simulink model "EMB"  (R2019b)
settings: Solver=ode45  StartTime=0.0  StopTime=1  RelTol=1e-3  EnableMultiTasking=on
values from neighbouring files (symbols this model uses):
  a = [1 10501 408092434.54 2.46403599001e+12 1.14030432406e+15 10480.8559648]    [EMB_Variables.mat]
  b = 4e+12    [EMB_Variables.mat]
  c_break = 1000000    [EMB_Variables.mat]
  c_gear = 200000    [EMB_Variables.mat]
  D_Kraft = 0    [EMB_Variables.mat]
  D_Pos = 0    [EMB_Variables.mat]
  d_rot = 0.1    [EMB_Variables.mat]
  d_trans = 0.1    [EMB_Variables.mat]
  i = 113.116658706    [EMB_Variables.mat]
  I_Kraft = 1000    [EMB_Variables.mat]
  I_Pos = 1000    [EMB_Variables.mat]
  J = 1e-05    [EMB_Variables.mat]
  K = 0.02    [EMB_Variables.mat]
  L = 0.001    [EMB_Variables.mat]
  m = 0.1    [EMB_Variables.mat]
  P_Kraft = 10000    [EMB_Variables.mat]
  P_Pos = 10000    [EMB_Variables.mat]
  R = 0.5    [EMB_Variables.mat]
  t0 = 0.1    [EMB_Variables.mat]
  t1 = 0.0025    [EMB_Variables.mat]
  T_abtast = 0.0001    [EMB_Variables.mat]
  x0 = 0.05    [EMB_Variables.mat]
  x_break = 0.0005    [EMB_Variables.mat]
libraries: simulink x3
settings Model: Creator=thomasst  LastModifiedBy=yuxia
settings DataIOCC: SaveFormat=Array  SignalLoggingSaveFormat=ModelDataLogs  ReturnWorkspaceOutputs=off
settings OptimizationCC: LifeSpan=inf
settings DebuggingCC: SolverPrmCheckMsg=warning  MultiTaskDSMMsg=warning  MultiTaskCondExecSysMsg=none  SFUnexpectedBacktrackingDiag=warning  SFNoUnconditionalDefaultTransitionDiag=warning  SFExecutionAtInitializationDiag=none  ArithmeticOperatorsInVariantConditions=warning
settings HardwareCC: ProdBitPerPointer=32  ProdBitPerSizeT=32  ProdBitPerPtrDiffT=32  ProdLargestAtomicFloat=None  ProdIntDivRoundTo=Undefined  ProdEndianess=Unspecified  ProdWordSize=32  ProdHWDeviceType=32-bit Generic
settings ModelReferenceCC: PropagateSignalLabelsOutOfModel=off
settings SFSimCC: SimUseLocalCustomCode=off  CustomCodeUndefinedFunction=UseInterfaceOnly
settings RTWCC: RTWUseLocalCustomCode=off
settings CodeAppCC: StateflowObjectComments=on
settings GRTTargetCC: TargetLangStandard=C89/C90 (ANSI)  GeneratePreprocessorConditionals=Disable all
settings ConfigComp: CovMetricSettings=dw  CovHtmlReporting=on  CovSaveCumulativeToWorkspaceVar=on  CovSaveSingleToWorkspaceVar=on  CovExternalEMLEnable=off

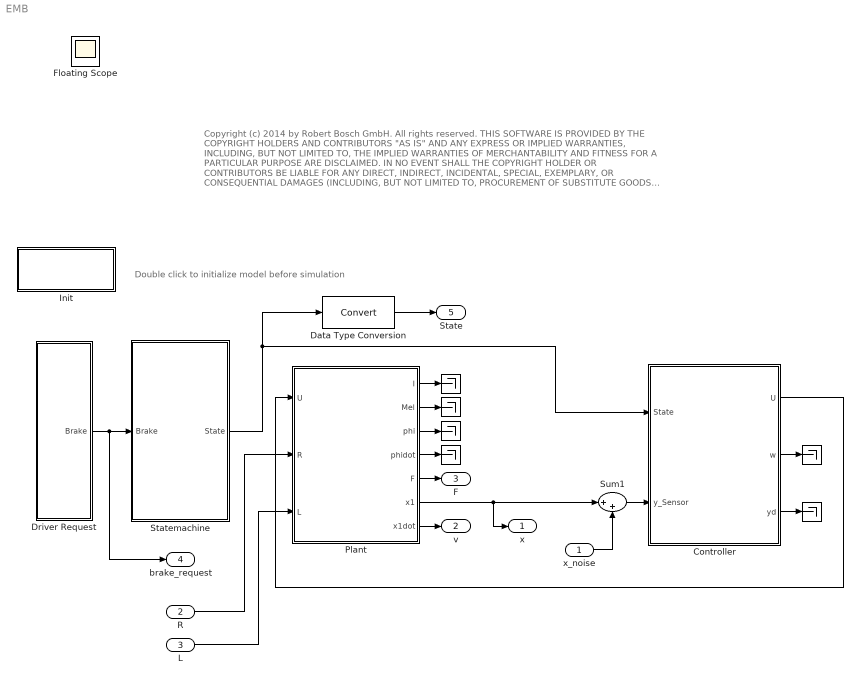
== system EMB ==
  note: Copyright (c) 2014 by Robert Bosch GmbH. All rights reserved.
      |
      | THIS SOFTWARE IS PROVIDED BY THE COPYRIGHT HOLDERS AND CONTRIBUTORS "AS IS"
      | AND ANY EXPRESS OR IMPLIED WARRANTIES, INCLUDING, BUT NOT LIMITED TO, THE IMPLIED
      | WARRANTIES OF MERCHANTABILITY AND FITNESS FOR A PARTICULAR PURPOSE ARE
      | DISCLAIMED. IN NO EVENT SHALL THE COPYRIGHT HOLDER OR CONTRIBUTORS BE LIABLE FOR
      | ANY DIRECT, INDIRECT, INCIDENTAL, SPECIAL, EXEMPLARY, OR CONSEQUENTIAL DAMAGES
      |  (INCLUDING, BUT NOT LIMITED TO, PROCUREMENT OF SUBSTITUTE GOODS OR SERVICES;
      | LOSS OF USE, DATA, OR PROFITS; OR BUSINESS INTERRUPTION) HOWEVER CAUSED AND
      | ON ANY THEORY OF LIABILITY, WHETHER IN CONTRACT, STRICT LIABILITY, OR TORT (INCLUDING
      | NEGLIGENCE OR OTHERWISE) ARISING IN ANY WAY OUT OF THE USE OF THIS SOFTWARE, EVEN
      | IF ADVISED OF THE POSSIBILITY OF SUCH DAMAGE.
      |
      | THE ENTIRE RISK AS TO THE QUALITY AND PERFORMANCE OF THE PROGRAM IS WITH YOU. SHOULD THE PROGRAM PROVE DEFECTIVE,
      | YOU ASSUME THE COST OF ALL NECESSARY SERVICING, REPAIR OR CORRECTION.
      |
      | This is not a model of a Bosch product.
      | This model was originally released in the scope of the ARCH workshop (http://cps-vo.org/group/ARCH).
  note: Double click to initialize model before simulation
  x_noise : Inport
  R : Inport  Port=2
  L : Inport  Port=3
  "  " : Terminator
  "   " : Terminator
  "    " : Terminator
  "      " : Terminator
  "        " : Terminator
  "          " : Terminator
  Controller : Subsystem
  Data Type Conversion : DataTypeConversion
  Driver Request : Subsystem
  Init : Subsystem
      settings: OpenFcn=load('EMB_Variables.mat');
  Plant : Subsystem
  Statemachine : Subsystem
  Sum1 : Sum  Inputs=|++
  x : Outport
  v : Outport  Port=2
  F : Outport  Port=3
  brake_request : Outport  Port=4
  State : Outport  Port=5
  Floating Scope : Scope
  wires:
  Plant/6(x1) -> Sum1/1, x/1
  Plant/3(phi) -> "  "/1
  Plant/4(phidot) -> "   "/1
  Plant/5(F) -> F/1
  Plant/7(x1dot) -> v/1
  x_noise/1 -> Sum1/2
  Plant/2(Mel) -> "    "/1
  Plant/1(I) -> "      "/1
  Sum1/1 -> Controller/2(y_Sensor)
  Controller/1(U) -> Plant/1(U)
  Controller/2(w) -> "          "/1
  Controller/3(yd) -> "        "/1
  Statemachine/1(State) -> Controller/1(State), Data Type Conversion/1
  Driver Request/1(Brake) -> Statemachine/1(Brake), brake_request/1
  Data Type Conversion/1 -> State/1
  R/1 -> Plant/2(R)
  L/1 -> Plant/3(L)

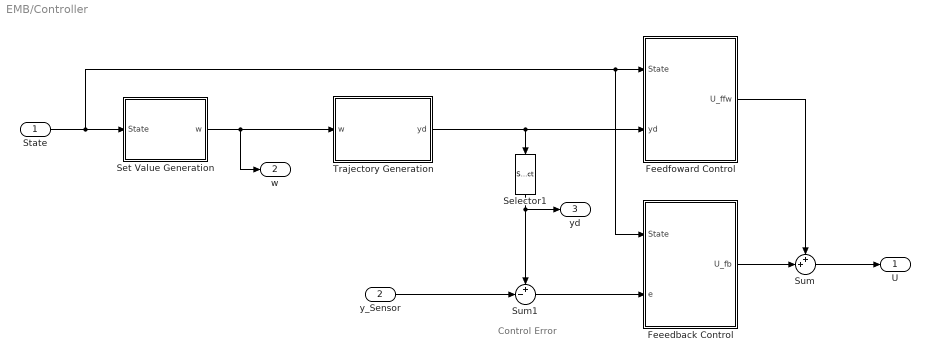
== system EMB/Controller ==
  note: Control Error
  State : Inport
  y_Sensor : Inport  Port=2
  Feedfoward Control : Subsystem
  Feeedback Control : Subsystem
  Selector1 : Selector  InputPortWidth=6  IndexOptions=Index vector (dialog)  Indices=[1]  OutputSizes=1
  Set Value Generation : Subsystem
  Sum : Sum  Inputs=++|
  Sum1 : Sum  Inputs=+-|
  Trajectory Generation : Subsystem
  U : Outport
  w : Outport  Port=2
  yd : Outport  Port=3
  wires:
  State/1 -> Set Value Generation/1(State), Feedfoward Control/1(State), Feeedback Control/1(State)
  Set Value Generation/1(w) -> Trajectory Generation/1(w), w/1
  Trajectory Generation/1(yd) -> Feedfoward Control/2(yd), Selector1/1
  Feedfoward Control/1(U_ffw) -> Sum/1
  Sum/1 -> U/1
  Feeedback Control/1(U_fb) -> Sum/2
  Sum1/1 -> Feeedback Control/2(e)
  Selector1/1 -> Sum1/1, yd/1
  y_Sensor/1 -> Sum1/2

== system EMB/Driver Request ==
  Pulse Generator : DiscretePulseGenerator  PulseType=Time based  Period=1  PulseWidth=50  PhaseDelay=0.01
  Brake : Outport
  wires:
  Pulse Generator/1 -> Brake/1

== system EMB/Init ==

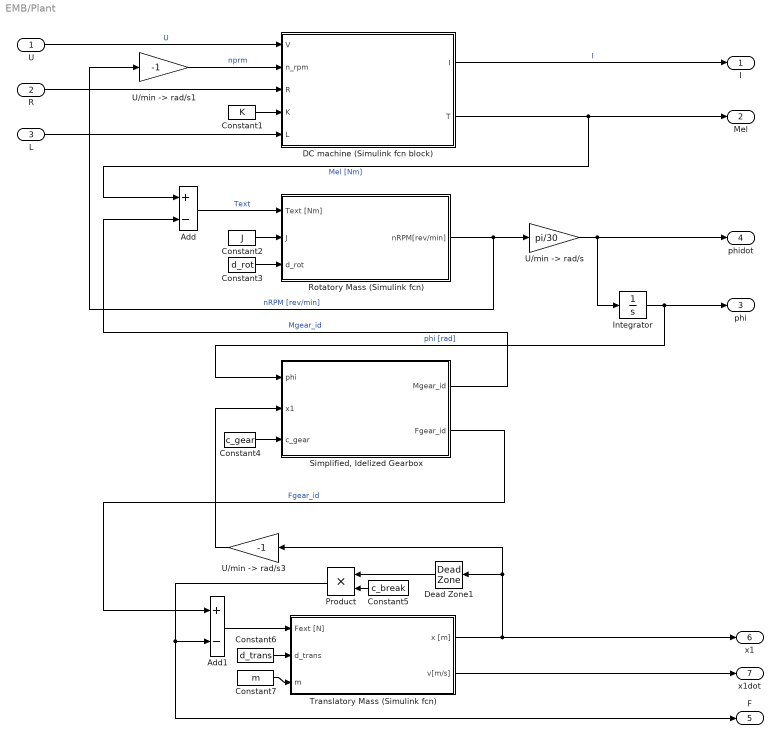
== system EMB/Plant ==
  U : Inport
  R : Inport  Port=2
  L : Inport  Port=3
  Add : Sum  Inputs=+-
  Add1 : Sum  Inputs=+-
  Constant1 : Constant  Value=K
  Constant2 : Constant  Value=J
  Constant3 : Constant  Value=d_rot
  Constant4 : Constant  Value=c_gear
  Constant5 : Constant  Value=c_break
  Constant6 : Constant  Value=d_trans
  Constant7 : Constant  Value=m
  DC machine (Simulink fcn block) : Subsystem
  Dead Zone1 : DeadZone  LowerValue=-inf  UpperValue=x0  SaturateOnIntegerOverflow=on
  Integrator : Integrator
  Product : Product
  Rotatory Mass (Simulink fcn) : Subsystem
  "Simplified, Idelized Gearbox" : Subsystem
  Translatory Mass (Simulink fcn) : Subsystem
  "U/min -> rad/s" : Gain  Gain=pi/30
  "U/min -> rad/s1" : Gain  Gain=-1
  "U/min -> rad/s3" : Gain  Gain=-1
  I : Outport
  Mel : Outport  Port=2
  phi : Outport  Port=3
  phidot : Outport  Port=4
  F : Outport  Port=5
  x1 : Outport  Port=6
  x1dot : Outport  Port=7
  wires:
  U/1 -> DC machine (Simulink fcn block)/1(V)  "U"
  "U/min -> rad/s1"/1 -> DC machine (Simulink fcn block)/2(n_rpm)  "nprm"
  Product/1 -> F/1, Add1/2
  Dead Zone1/1 -> Product/1
  "U/min -> rad/s3"/1 -> "Simplified, Idelized Gearbox"/2(x1)
  "Simplified, Idelized Gearbox"/2(Fgear_id) -> Add1/1  "Fgear_id"
  "Simplified, Idelized Gearbox"/1(Mgear_id) -> Add/2  "Mgear_id"
  DC machine (Simulink fcn block)/2(T) -> Mel/1, Add/1  "Mel [Nm]"
  Translatory Mass (Simulink fcn)/1(x [m]) -> Dead Zone1/1, "U/min -> rad/s3"/1, x1/1
  Add1/1 -> Translatory Mass (Simulink fcn)/1(Fext [N])
  Integrator/1 -> phi/1, "Simplified, Idelized Gearbox"/1(phi)  "phi [rad]"
  "U/min -> rad/s"/1 -> Integrator/1, phidot/1
  Rotatory Mass (Simulink fcn)/1(nRPM[rev/min]) -> "U/min -> rad/s"/1, "U/min -> rad/s1"/1  "nRPM [rev/min]"
  Add/1 -> Rotatory Mass (Simulink fcn)/1(Text [Nm])  "Text"
  DC machine (Simulink fcn block)/1(I) -> I/1  "I"
  Translatory Mass (Simulink fcn)/2(v[m/s]) -> x1dot/1
  R/1 -> DC machine (Simulink fcn block)/3(R)
  Constant1/1 -> DC machine (Simulink fcn block)/4(K)
  L/1 -> DC machine (Simulink fcn block)/5(L)
  Constant2/1 -> Rotatory Mass (Simulink fcn)/2(J)
  Constant3/1 -> Rotatory Mass (Simulink fcn)/3(d_rot)
  Constant4/1 -> "Simplified, Idelized Gearbox"/3(c_gear)
  Constant5/1 -> Product/2
  Constant6/1 -> Translatory Mass (Simulink fcn)/2(d_trans)
  Constant7/1 -> Translatory Mass (Simulink fcn)/3(m)

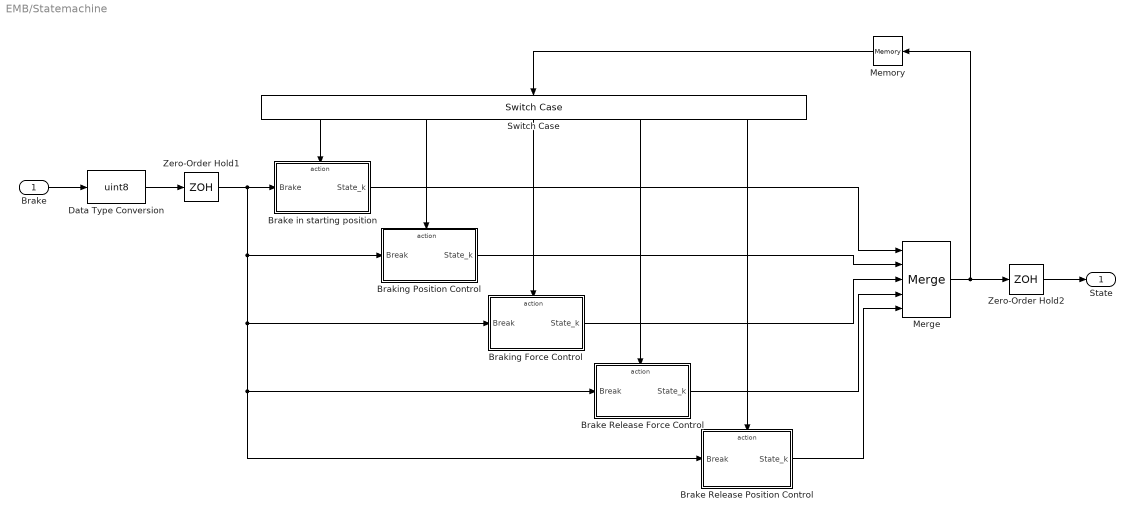
== system EMB/Statemachine ==
  Brake : Inport
  Brake Release Force Control : Subsystem  TreatAsAtomicUnit=on
  Brake Release Position Control : Subsystem  TreatAsAtomicUnit=on
  Brake in starting position : Subsystem  TreatAsAtomicUnit=on
  Braking Force Control : Subsystem  TreatAsAtomicUnit=on
  Braking Position Control : Subsystem  TreatAsAtomicUnit=on
  Data Type Conversion : DataTypeConversion  OutDataTypeStr=uint8
  Memory : Memory  InheritSampleTime=on
  Merge : Merge  Inputs=5
  Switch Case : SwitchCase  CaseConditions={0,1,2,3,4}  ShowDefaultCase=off
  Zero-Order Hold1 : ZeroOrderHold  SampleTime=T_abtast
  Zero-Order Hold2 : ZeroOrderHold  SampleTime=T_abtast
  State : Outport
  wires:
  Merge/1 -> Memory/1, Zero-Order Hold2/1
  Memory/1 -> Switch Case/1
  Zero-Order Hold1/1 -> Brake in starting position/1(Brake), Braking Position Control/1(Break), Braking Force Control/1(Break), Brake Release Force Control/1(Break), Brake Release Position Control/1(Break)
  Switch Case/1 -> Brake in starting position/Action
  Switch Case/2 -> Braking Position Control/Action
  Switch Case/3 -> Braking Force Control/Action
  Switch Case/4 -> Brake Release Force Control/Action
  Switch Case/5 -> Brake Release Position Control/Action
  Brake in starting position/1(State_k) -> Merge/1
  Braking Position Control/1(State_k) -> Merge/2
  Braking Force Control/1(State_k) -> Merge/3
  Brake Release Force Control/1(State_k) -> Merge/4
  Brake Release Position Control/1(State_k) -> Merge/5
  Zero-Order Hold2/1 -> State/1
  Data Type Conversion/1 -> Zero-Order Hold1/1
  Brake/1 -> Data Type Conversion/1

== system EMB/Controller/Feedfoward Control ==
  State : Inport
  yd : Inport  Port=2
  Constant : Constant  Value=0
  Demux : Demux  Outputs=6
  Feedforward Control Force : S-Function  FunctionName=InverseEMBforce  Parameters=R,L,K,J,dvrot,m,dvtrans,cgear,i,cbreak,x0,xic  SFunctionDeploymentMode=off  EnableBusSupport=off  mask{R=R, L=L, K=K, J=J, dvrot=d_rot, m=m, dvtrans=d_trans, cgear=c_gear, i=i, cbreak=c_break, x0=x0, xic=[0]}
      mask prompts: R "Widerstand R [Ohm]:"; L "Induktivitaet L [H]:"; K "Motorkonstante K [Vs]:"; J "Traegheitsmoment J [kgm^2]:"; dvrot "Viskose Reibung dvrot [Nms/rad]:"; m "Masse m [kg]:"; dvtrans "Viskose Reibung dvtrans [Ns/m]:"; cgear "Steifigkeit Getriebe cgear [N/m]:"; i "Uebersetzung i [-]:"; cbreak "Steifigkeit Bremse cbreak [N/m]:"; x0 "Position x0 [m]:"; xic "Vector of continuous initial conditions [Initial Dummy]"
  Feedforward Control Position : Fcn  Expr="(a(1)*u[6] + a(2)*u[5] + a(3)*u[4] + a(4)*u[3]  + a(5)*u[2] + a(6)*u[1] )/b"
  Multiport Switch : MultiPortSwitch  DataPortOrder=Zero-based contiguous  Inputs=5  zeroidx=on
  U_ffw : Outport
  wires:
  State/1 -> Multiport Switch/1
  yd/1 -> Feedforward Control Position/1, Demux/1
  Demux/1 -> Feedforward Control Force/1
  Demux/2 -> Feedforward Control Force/2
  Demux/3 -> Feedforward Control Force/3
  Demux/4 -> Feedforward Control Force/4
  Demux/5 -> Feedforward Control Force/5
  Demux/6 -> Feedforward Control Force/6
  Constant/1 -> Multiport Switch/2
  Feedforward Control Position/1 -> Multiport Switch/3, Multiport Switch/6
  Feedforward Control Force/1 -> Multiport Switch/4, Multiport Switch/5
  Multiport Switch/1 -> U_ffw/1

== system EMB/Controller/Feeedback Control ==
  State : Inport
  e : Inport  Port=2
  Brakin in starting Position : Subsystem  TreatAsAtomicUnit=on
  Force Control : Subsystem  TreatAsAtomicUnit=on
  Multiport Switch : MultiPortSwitch  DataPortOrder=Zero-based contiguous  Inputs=5  zeroidx=on
  Position Control : Subsystem  TreatAsAtomicUnit=on
  Switch Case : SwitchCase  CaseConditions={0,[1,4],[2,3]}  ShowDefaultCase=off  SampleTime=T_abtast
  U_fb : Outport
  wires:
  State/1 -> Switch Case/1, Multiport Switch/1
  Switch Case/1 -> Brakin in starting Position/Action
  e/1 -> Position Control/1(e), Force Control/1(e)
  Switch Case/2 -> Position Control/Action
  Switch Case/3 -> Force Control/Action
  Position Control/1(U) -> Multiport Switch/3, Multiport Switch/6
  Brakin in starting Position/1(U) -> Multiport Switch/2
  Force Control/1(U) -> Multiport Switch/4, Multiport Switch/5
  Multiport Switch/1 -> U_fb/1

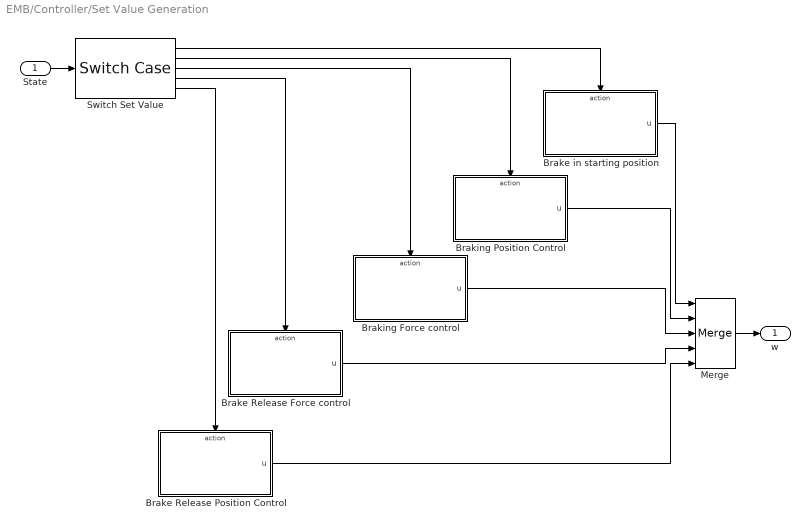
== system EMB/Controller/Set Value Generation ==
  State : Inport
  Brake Release Force control : Subsystem  TreatAsAtomicUnit=on
  Brake Release Position Control : Subsystem  TreatAsAtomicUnit=on
  Brake in starting position : Subsystem  TreatAsAtomicUnit=on
  Braking Force control : Subsystem  TreatAsAtomicUnit=on
  Braking Position Control : Subsystem  TreatAsAtomicUnit=on
  Merge : Merge  Inputs=5
  Switch Set Value : SwitchCase  CaseConditions={0,1,2,3,4}  ShowDefaultCase=off
  w : Outport
  wires:
  Switch Set Value/1 -> Brake in starting position/Action
  Brake in starting position/1(u) -> Merge/1
  Switch Set Value/2 -> Braking Position Control/Action
  Braking Position Control/1(u) -> Merge/2
  Switch Set Value/3 -> Braking Force control/Action
  Switch Set Value/4 -> Brake Release Force control/Action
  Braking Force control/1(u) -> Merge/3
  Brake Release Force control/1(u) -> Merge/4
  Switch Set Value/5 -> Brake Release Position Control/Action
  Brake Release Position Control/1(u) -> Merge/5
  State/1 -> Switch Set Value/1
  Merge/1 -> w/1

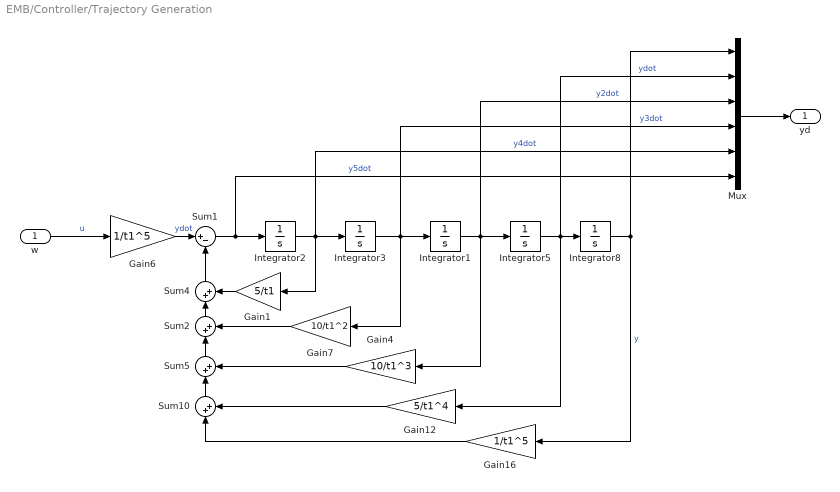
== system EMB/Controller/Trajectory Generation ==
  w : Inport
  Gain1 : Gain  Gain=5/t1
  Gain12 : Gain  Gain=5/t1^4
  Gain16 : Gain  Gain=1/t1^5
  Gain4 : Gain  Gain=10/t1^3
  Gain6 : Gain  Gain=1/t1^5
  Gain7 : Gain  Gain=10/t1^2
  Integrator{1..3,5,8} (5 alike) : Integrator
  Mux : Mux  Inputs=6
  Sum1 : Sum  Inputs=|+-
  Sum{2,4..5,10} (4 alike) : Sum  Inputs=|++
  yd : Outport
  wires:
  w/1 -> Gain6/1  "u"
  Mux/1 -> yd/1
  Integrator2/1 -> Gain1/1, Mux/5, Integrator3/1  "y4dot"
  Sum1/1 -> Integrator2/1, Mux/6  "y5dot"
  Gain6/1 -> Sum1/1  "ydot"
  Integrator3/1 -> Gain7/1, Mux/4, Integrator1/1  "y3dot"
  Gain7/1 -> Sum2/2
  Integrator1/1 -> Gain4/1, Mux/3, Integrator5/1  "y2dot"
  Gain4/1 -> Sum5/2
  Sum4/1 -> Sum1/2
  Gain1/1 -> Sum4/2
  Sum2/1 -> Sum4/1
  Integrator5/1 -> Gain12/1, Mux/2, Integrator8/1  "ydot"
  Sum5/1 -> Sum2/1
  Integrator8/1 -> Gain16/1, Mux/1  "y"
  Gain12/1 -> Sum10/2
  Sum10/1 -> Sum5/1
  Gain16/1 -> Sum10/1

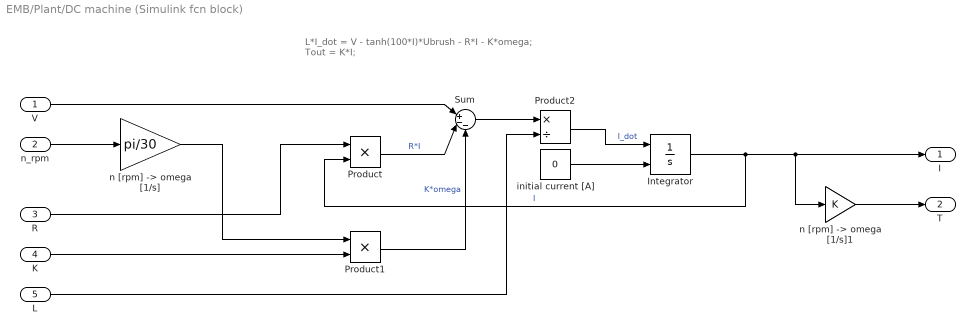
== system EMB/Plant/DC machine (Simulink fcn block) ==
  note: L*I_dot = V - tanh(100*I)*Ubrush - R*I - K*omega;
      | Tout = K*I;
  V : Inport
  n_rpm : Inport  Port=2
  R : Inport  Port=3
  K : Inport  Port=4
  L : Inport  Port=5
  Integrator : Integrator  InitialConditionSource=external
  Product : Product
  Product1 : Product
  Product2 : Product  Inputs=*/
  Sum : Sum  Inputs=|+--
  initial current [A] : Constant  Value=0
  "n [rpm] -> omega [1/s]" : Gain  Gain=pi/30
  "n [rpm] -> omega [1/s]1" : Gain  Gain=K
  I : Outport
  T : Outport  Port=2
  wires:
  n_rpm/1 -> "n [rpm] -> omega [1/s]"/1
  V/1 -> Sum/1
  "n [rpm] -> omega [1/s]"/1 -> Product1/1
  "n [rpm] -> omega [1/s]1"/1 -> T/1
  Product2/1 -> Integrator/1  "I_dot"
  Integrator/1 -> Product/2, I/1, "n [rpm] -> omega [1/s]1"/1  "I"
  initial current [A]/1 -> Integrator/2
  R/1 -> Product/1
  Product/1 -> Sum/2  "R*I"
  Product1/1 -> Sum/3  "K*omega"
  K/1 -> Product1/2
  L/1 -> Product2/2
  Sum/1 -> Product2/1

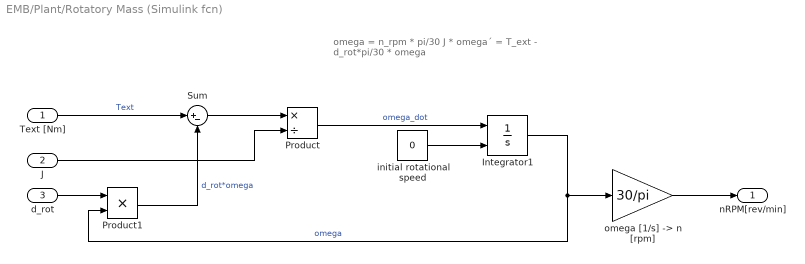
== system EMB/Plant/Rotatory Mass (Simulink fcn) ==
  note: omega = n_rpm * pi/30
      |
      | J * omega´ = T_ext -  d_rot*pi/30 * omega
  Text [Nm] : Inport
  J : Inport  Port=2
  d_rot : Inport  Port=3
  Integrator1 : Integrator  InitialConditionSource=external
  Product : Product  Inputs=*/
  Product1 : Product
  Sum : Sum  Inputs=|+-
  initial rotational speed : Constant  Value=0
  "omega [1/s] -> n [rpm]" : Gain  Gain=30/pi
  nRPM[rev/min] : Outport
  wires:
  "omega [1/s] -> n [rpm]"/1 -> nRPM[rev/min]/1
  Product/1 -> Integrator1/1  "omega_dot"
  initial rotational speed/1 -> Integrator1/2
  Integrator1/1 -> Product1/2, "omega [1/s] -> n [rpm]"/1  "omega"
  J/1 -> Product/2
  Product1/1 -> Sum/2  "d_rot*omega"
  Text [Nm]/1 -> Sum/1  "Text"
  d_rot/1 -> Product1/1
  Sum/1 -> Product/1

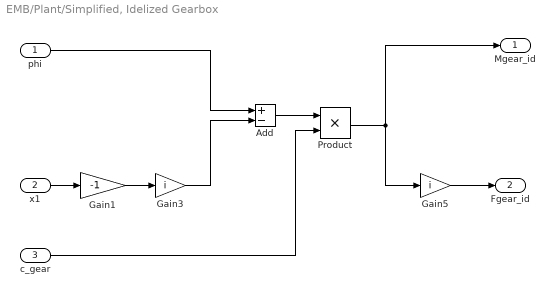
== system EMB/Plant/Simplified, Idelized Gearbox ==
  phi : Inport
  x1 : Inport  Port=2
  c_gear : Inport  Port=3
  Add : Sum  Inputs=+-
  Gain1 : Gain  Gain=-1
  Gain3 : Gain  Gain=i
  Gain5 : Gain  Gain=i
  Product : Product
  Mgear_id : Outport
  Fgear_id : Outport  Port=2
  wires:
  Gain1/1 -> Gain3/1
  x1/1 -> Gain1/1
  Gain5/1 -> Fgear_id/1
  Product/1 -> Mgear_id/1, Gain5/1
  Add/1 -> Product/1
  Gain3/1 -> Add/2
  phi/1 -> Add/1
  c_gear/1 -> Product/2

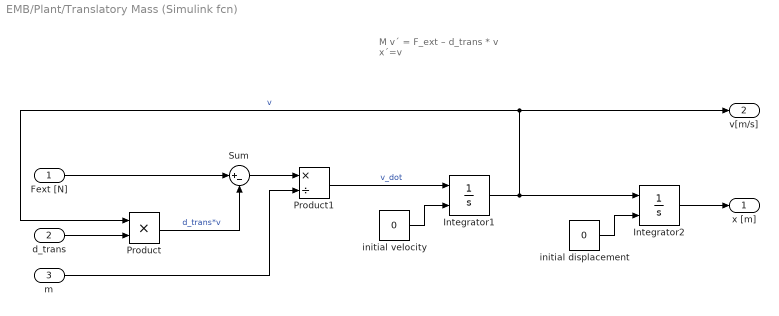
== system EMB/Plant/Translatory Mass (Simulink fcn) ==
  note: M v´ = F_ext – d_trans * v
      |
      | x´=v
  Fext [N] : Inport
  d_trans : Inport  Port=2
  m : Inport  Port=3
  Integrator1 : Integrator  InitialConditionSource=external
  Integrator2 : Integrator  InitialConditionSource=external
  Product : Product
  Product1 : Product  Inputs=*/
  Sum : Sum  Inputs=|+-
  initial displacement : Constant  Value=0
  "initial velocity " : Constant  Value=0
  x [m] : Outport
  v[m/s] : Outport  Port=2
  wires:
  initial displacement/1 -> Integrator2/2
  Fext [N]/1 -> Sum/1
  Integrator1/1 -> v[m/s]/1, Product/1, Integrator2/1  "v"
  "initial velocity "/1 -> Integrator1/2
  Product1/1 -> Integrator1/1  "v_dot"
  Integrator2/1 -> x [m]/1
  d_trans/1 -> Product/2
  Product/1 -> Sum/2  "d_trans*v"
  Sum/1 -> Product1/1
  m/1 -> Product1/2

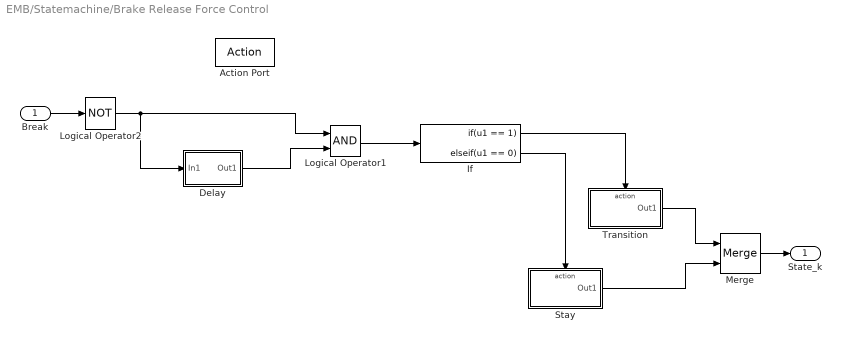
== system EMB/Statemachine/Brake Release Force Control ==
  Break : Inport
  Action Port : ActionPort  InitializeStates=reset  ActionPortLabel=case [ 3 ]:
  Delay : Subsystem
  If : If  IfExpression=u1 == 1  ElseIfExpressions=u1 == 0  ShowElse=off
  Logical Operator1 : Logic  AllPortsSameDT=off  OutDataTypeStr=boolean
  Logical Operator2 : Logic  Operator=NOT  AllPortsSameDT=off  OutDataTypeStr=boolean
  Merge : Merge
  Stay : Subsystem  TreatAsAtomicUnit=on
  Transition : Subsystem  TreatAsAtomicUnit=on
  State_k : Outport
  wires:
  Merge/1 -> State_k/1
  Stay/1(Out1) -> Merge/2
  Transition/1(Out1) -> Merge/1
  If/2 -> Stay/Action
  If/1 -> Transition/Action
  Break/1 -> Logical Operator2/1
  Logical Operator1/1 -> If/1
  Logical Operator2/1 -> Logical Operator1/1, Delay/1(In1)
  Delay/1(Out1) -> Logical Operator1/2

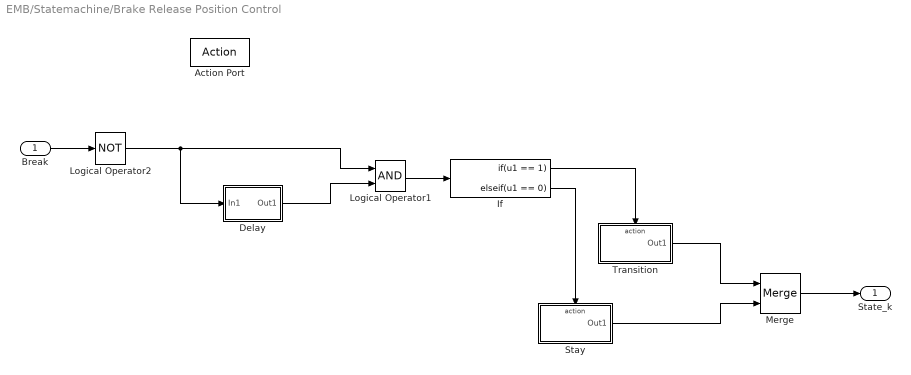
== system EMB/Statemachine/Brake Release Position Control ==
  Break : Inport
  Action Port : ActionPort  InitializeStates=reset  ActionPortLabel=case [ 4 ]:
  Delay : Subsystem
  If : If  IfExpression=u1 == 1  ElseIfExpressions=u1 == 0  ShowElse=off
  Logical Operator1 : Logic  AllPortsSameDT=off  OutDataTypeStr=boolean
  Logical Operator2 : Logic  Operator=NOT  AllPortsSameDT=off  OutDataTypeStr=boolean
  Merge : Merge
  Stay : Subsystem  TreatAsAtomicUnit=on
  Transition : Subsystem  TreatAsAtomicUnit=on
  State_k : Outport
  wires:
  Merge/1 -> State_k/1
  Stay/1(Out1) -> Merge/2
  Transition/1(Out1) -> Merge/1
  If/2 -> Stay/Action
  If/1 -> Transition/Action
  Break/1 -> Logical Operator2/1
  Logical Operator1/1 -> If/1
  Logical Operator2/1 -> Logical Operator1/1, Delay/1(In1)
  Delay/1(Out1) -> Logical Operator1/2

== system EMB/Statemachine/Brake in starting position ==
  Brake : Inport
  Action Port : ActionPort  ActionPortLabel=case [ 0 ]:
  If : If  IfExpression=u1 == 1  ElseIfExpressions=u1 == 0  ShowElse=off
  Merge : Merge
  Stay : Subsystem  TreatAsAtomicUnit=on
  Transition : Subsystem  TreatAsAtomicUnit=on
  State_k : Outport
  wires:
  Brake/1 -> If/1
  If/1 -> Transition/Action
  If/2 -> Stay/Action
  Transition/1(Out1) -> Merge/1
  Stay/1(Out1) -> Merge/2
  Merge/1 -> State_k/1

== system EMB/Statemachine/Braking Force Control ==
  Break : Inport
  Action Port : ActionPort  ActionPortLabel=case [ 2 ]:
  If : If  IfExpression=u1 == 0  ElseIfExpressions=u1 == 1  ShowElse=off
  Merge : Merge
  Stay : Subsystem  TreatAsAtomicUnit=on
  Transition : Subsystem  TreatAsAtomicUnit=on
  State_k : Outport
  wires:
  Merge/1 -> State_k/1
  Stay/1(Out1) -> Merge/2
  Transition/1(Out1) -> Merge/1
  If/2 -> Stay/Action
  If/1 -> Transition/Action
  Break/1 -> If/1

== system EMB/Statemachine/Braking Position Control ==
  Break : Inport
  Action Port : ActionPort  InitializeStates=reset  ActionPortLabel=case [ 1 ]:
  Delay : Subsystem
  If : If  IfExpression=u1 == 1  ElseIfExpressions=u1 == 0  ShowElse=off
  Logical Operator : Logic  AllPortsSameDT=off  OutDataTypeStr=boolean
  Merge : Merge
  Stay : Subsystem  TreatAsAtomicUnit=on
  Transition : Subsystem  TreatAsAtomicUnit=on
  State_k : Outport
  wires:
  If/1 -> Transition/Action
  If/2 -> Stay/Action
  Transition/1(Out1) -> Merge/1
  Stay/1(Out1) -> Merge/2
  Merge/1 -> State_k/1
  Break/1 -> Logical Operator/1, Delay/1(In1)
  Logical Operator/1 -> If/1
  Delay/1(Out1) -> Logical Operator/2

== system EMB/Controller/Feeedback Control/Brakin in starting Position ==
  Action Port : ActionPort  ActionPortLabel=case [ 0 ]:
  Constant : Constant  Value=0
  U : Outport
  wires:
  Constant/1 -> U/1

== system EMB/Controller/Feeedback Control/Force Control ==
  e : Inport
  Action Port : ActionPort  InitializeStates=reset  ActionPortLabel=case [ 2 3 ]:
  Gain : Gain
  PIDT1 zeitdiskret : Subsystem
  U : Outport
  wires:
  Gain/1 -> U/1
  PIDT1 zeitdiskret/1(y) -> Gain/1
  e/1 -> PIDT1 zeitdiskret/1(u)

== system EMB/Controller/Feeedback Control/Position Control ==
  e : Inport
  Action Port : ActionPort  InitializeStates=reset  ActionPortLabel=case [ 1 4 ]:
  Gain : Gain
  PIDT1 zeitdiskret : Subsystem
  U : Outport
  wires:
  e/1 -> PIDT1 zeitdiskret/1(u)
  PIDT1 zeitdiskret/1(y) -> Gain/1
  Gain/1 -> U/1

== system EMB/Controller/Set Value Generation/Brake Release Force control ==
  Action Port : ActionPort  ActionPortLabel=case [ 3 ]:
  Constant : Constant  Value=x0
  u : Outport
  wires:
  Constant/1 -> u/1

== system EMB/Controller/Set Value Generation/Brake Release Position Control ==
  Action Port : ActionPort  ActionPortLabel=case [ 4 ]:
  Constant : Constant  Value=0
  u : Outport
  wires:
  Constant/1 -> u/1

== system EMB/Controller/Set Value Generation/Brake in starting position ==
  Action Port : ActionPort  ActionPortLabel=case [ 0 ]:
  Constant : Constant  Value=0
  u : Outport
  wires:
  Constant/1 -> u/1

== system EMB/Controller/Set Value Generation/Braking Force control ==
  Action Port : ActionPort  ActionPortLabel=case [ 2 ]:
  Constant : Constant  Value=x0 + x_break
  u : Outport
  wires:
  Constant/1 -> u/1

== system EMB/Controller/Set Value Generation/Braking Position Control ==
  Action Port : ActionPort  ActionPortLabel=case [ 1 ]:
  Constant : Constant  Value=x0
  u : Outport
  wires:
  Constant/1 -> u/1

== system EMB/Statemachine/Brake Release Force Control/Delay ==
  In1 : Inport
  Compare To Constant : simulink/Logic and Bit Operations/Compare To Constant  relop=>=  const=t0  OutDataTypeStr=uint8  ZeroCross=off
  Data Type Conversion : DataTypeConversion
  Integrator : Integrator
  Out1 : Outport
  wires:
  In1/1 -> Data Type Conversion/1
  Integrator/1 -> Compare To Constant/1
  Compare To Constant/1 -> Out1/1
  Data Type Conversion/1 -> Integrator/1

== system EMB/Statemachine/Brake Release Force Control/Stay ==
  Action Port : ActionPort  ActionPortLabel=elseif(u1 == 0)
  Constant : Constant  Value=3  OutDataTypeStr=uint8
  Out1 : Outport
  wires:
  Constant/1 -> Out1/1

== system EMB/Statemachine/Brake Release Force Control/Transition ==
  Action Port : ActionPort  ActionPortLabel=if(u1 == 1)
  Constant : Constant  Value=4  OutDataTypeStr=uint8
  Out1 : Outport
  wires:
  Constant/1 -> Out1/1

== system EMB/Statemachine/Brake Release Position Control/Delay ==
  In1 : Inport
  Compare To Constant : simulink/Logic and Bit Operations/Compare To Constant  relop=>=  const=t0  OutDataTypeStr=uint8  ZeroCross=off
  Data Type Conversion : DataTypeConversion
  Integrator : Integrator
  Out1 : Outport
  wires:
  In1/1 -> Data Type Conversion/1
  Integrator/1 -> Compare To Constant/1
  Compare To Constant/1 -> Out1/1
  Data Type Conversion/1 -> Integrator/1

== system EMB/Statemachine/Brake Release Position Control/Stay ==
  Action Port : ActionPort  ActionPortLabel=elseif(u1 == 0)
  Constant : Constant  Value=4  OutDataTypeStr=uint8
  Out1 : Outport
  wires:
  Constant/1 -> Out1/1

== system EMB/Statemachine/Brake Release Position Control/Transition ==
  Action Port : ActionPort  ActionPortLabel=if(u1 == 1)
  Constant : Constant  Value=0  OutDataTypeStr=uint8
  Out1 : Outport
  wires:
  Constant/1 -> Out1/1

== system EMB/Statemachine/Brake in starting position/Stay ==
  Action Port : ActionPort  ActionPortLabel=elseif(u1 == 0)
  Constant : Constant  Value=0  OutDataTypeStr=uint8
  Out1 : Outport
  wires:
  Constant/1 -> Out1/1

== system EMB/Statemachine/Brake in starting position/Transition ==
  Action Port : ActionPort  ActionPortLabel=if(u1 == 1)
  Constant : Constant  OutDataTypeStr=uint8
  Out1 : Outport
  wires:
  Constant/1 -> Out1/1

== system EMB/Statemachine/Braking Force Control/Stay ==
  Action Port : ActionPort  ActionPortLabel=elseif(u1 == 1)
  Constant : Constant  Value=2  OutDataTypeStr=uint8
  Out1 : Outport
  wires:
  Constant/1 -> Out1/1

== system EMB/Statemachine/Braking Force Control/Transition ==
  Action Port : ActionPort  ActionPortLabel=if(u1 == 0)
  Constant : Constant  Value=3  OutDataTypeStr=uint8
  Out1 : Outport
  wires:
  Constant/1 -> Out1/1

== system EMB/Statemachine/Braking Position Control/Delay ==
  In1 : Inport
  Compare To Constant : simulink/Logic and Bit Operations/Compare To Constant  relop=>=  const=t0  OutDataTypeStr=uint8  ZeroCross=off
  Data Type Conversion : DataTypeConversion
  Integrator : Integrator
  Out1 : Outport
  wires:
  In1/1 -> Data Type Conversion/1
  Integrator/1 -> Compare To Constant/1
  Compare To Constant/1 -> Out1/1
  Data Type Conversion/1 -> Integrator/1

== system EMB/Statemachine/Braking Position Control/Stay ==
  Action Port : ActionPort  ActionPortLabel=elseif(u1 == 0)
  Constant : Constant  OutDataTypeStr=uint8
  Out1 : Outport
  wires:
  Constant/1 -> Out1/1

== system EMB/Statemachine/Braking Position Control/Transition ==
  Action Port : ActionPort  ActionPortLabel=if(u1 == 1)
  Constant : Constant  Value=2  OutDataTypeStr=uint8
  Out1 : Outport
  wires:
  Constant/1 -> Out1/1

== system EMB/Controller/Feeedback Control/Force Control/PIDT1 zeitdiskret ==
  u : Inport
  Discrete Transfer Fcn : DiscreteTransferFcn  Numerator=[1 1]  Denominator=[1 -1]  SampleTime=T_abtast
  Discrete Transfer Fcn1 : DiscreteTransferFcn  Numerator=[1 -1]  Denominator=[1+1/tan(T_abtast/2/1e-3) 1-1/tan(T_abtast/2/1e-3)]  SampleTime=T_abtast
  Sum : Sum  Inputs=3
  proportinal part : Gain  Gain=P_Kraft
  proportinal part1 : Gain  Gain=I_Kraft*T_abtast/2
  proportinal part2 : Gain  Gain=2*D_Kraft/T_abtast
  y : Outport
  wires:
  Sum/1 -> y/1
  proportinal part/1 -> Sum/1
  u/1 -> proportinal part1/1, proportinal part2/1, proportinal part/1
  Discrete Transfer Fcn/1 -> Sum/2
  Discrete Transfer Fcn1/1 -> Sum/3
  proportinal part1/1 -> Discrete Transfer Fcn/1
  proportinal part2/1 -> Discrete Transfer Fcn1/1

== system EMB/Controller/Feeedback Control/Position Control/PIDT1 zeitdiskret ==
  u : Inport
  Discrete Transfer Fcn : DiscreteTransferFcn  Numerator=[1 1]  Denominator=[1 -1]  SampleTime=T_abtast
  Discrete Transfer Fcn1 : DiscreteTransferFcn  Numerator=[1 -1]  Denominator=[1+1/tan(T_abtast/2/1e-3) 1-1/tan(T_abtast/2/1e-3)]  SampleTime=T_abtast
  Sum : Sum  Inputs=3
  proportinal part : Gain  Gain=P_Pos
  proportinal part1 : Gain  Gain=I_Pos*T_abtast/2
  proportinal part2 : Gain  Gain=2*D_Pos/T_abtast
  y : Outport
  wires:
  Sum/1 -> y/1
  proportinal part/1 -> Sum/1
  u/1 -> proportinal part1/1, proportinal part2/1, proportinal part/1
  Discrete Transfer Fcn/1 -> Sum/2
  Discrete Transfer Fcn1/1 -> Sum/3
  proportinal part1/1 -> Discrete Transfer Fcn/1
  proportinal part2/1 -> Discrete Transfer Fcn1/1
